simulink model "simulacao_sem_linearizar2"  (R2017a)
settings: Solver=VariableStepAuto  StartTime=0.0  StopTime=50  RelTol=1e-3
values from neighbouring files (symbols this model uses):
  a = -9128    [prepare_y_prbs.m]
undefined symbols (not defined in the file or in its folder): g, m
settings Model: Creator=Mateus  LastModifiedBy=Mateus

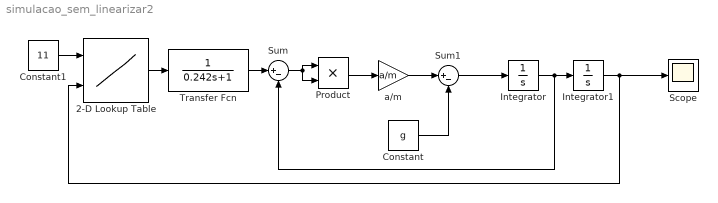
== system simulacao_sem_linearizar2 ==
  2-D Lookup Table : Lookup_n-D  BreakpointsForDimension1=[4,8,12,16]  BreakpointsForDimension2=[0,10,20,30,40,50,60,70,80]  Table=reshape([6.1,12,16.1,19.8,5.8,10.5,14.5,18,5.7,10,13,16.5,5,9,11.6,14,4.3,8,11,13,4.2,7.3,9.5,11,4,6.2,9,10,3.7,5.5,8,9,1,4.3,6.5,6.5],4,9)  InternalRulePriority=Speed  RndMeth=Simplest  InputSameDT=on
  Constant : Constant  Value=g
  Constant1 : Constant  Value=11
  Integrator : Integrator
  Integrator1 : Integrator  InitialCondition=0.2
  Product : Product
  Scope : Scope
  Sum : Sum  Inputs=|+-
  Sum1 : Sum  Inputs=|+-
  Transfer Fcn : TransferFcn  Denominator=[0.242 1]
  a/m : Gain  Gain=a/m
  wires:
  Integrator/1 -> Sum/2, Integrator1/1
  Integrator1/1 -> Scope/1, 2-D Lookup Table/2
  Sum/1 -> Product/1, Product/2
  Product/1 -> a/m/1
  a/m/1 -> Sum1/1
  Sum1/1 -> Integrator/1
  Constant/1 -> Sum1/2
  2-D Lookup Table/1 -> Transfer Fcn/1
  Transfer Fcn/1 -> Sum/1
  Constant1/1 -> 2-D Lookup Table/1
